simulink model "simulacaoEKF"  (R2016a)
settings: Solver=ode45  StartTime=0.0  StopTime=tf  RelTol=1e-3
undefined symbols (not defined in the file): x0
settings Model: Creator=Davi  LastModifiedBy=davia
settings DataIOCC: LimitDataPoints=on  SaveFormat=Array
settings HardwareCC: ProdBitPerPointer=32  ProdLargestAtomicFloat=None  ProdIntDivRoundTo=Undefined  ProdEndianess=Unspecified  ProdWordSize=32  ProdHWDeviceType=32-bit Generic
settings ModelReferenceCC: PropagateSignalLabelsOutOfModel=off
settings ConfigComp: CovModelRefEnable=Off

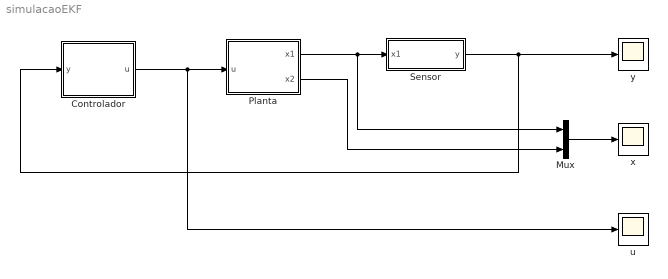
== system simulacaoEKF ==
  Controlador : Subsystem
  Mux : Mux  Inputs=2
  Planta : Subsystem
  "Sensor " : Subsystem
  u : Scope
  x : Scope
  y : Scope
  wires:
  Controlador/1(u) -> u/1, Planta/1(u)
  Planta/1(x1) -> Mux/1, "Sensor "/1(x1)
  "Sensor "/1(y) -> y/1, Controlador/1(y)
  Mux/1 -> x/1
  Planta/2(x2) -> Mux/2

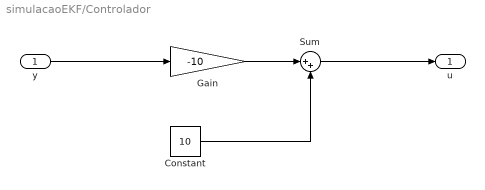
== system simulacaoEKF/Controlador ==
  y : Inport
  Constant : Constant  Value=10
  Gain : Gain  Gain=-10
  Sum : Sum  Inputs=|++
  u : Outport
  wires:
  y/1 -> Gain/1
  Constant/1 -> Sum/2
  Gain/1 -> Sum/1
  Sum/1 -> u/1

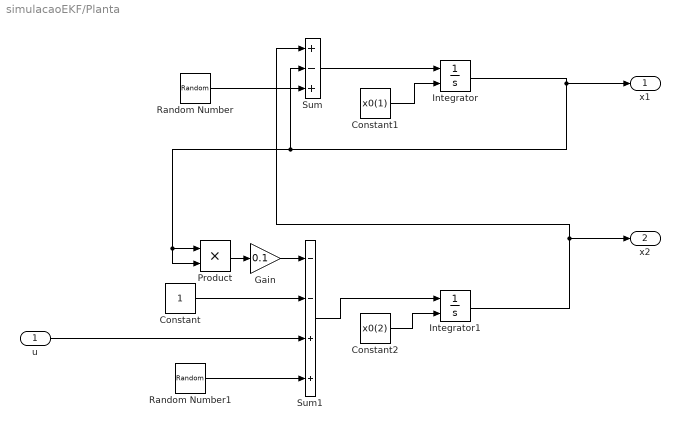
== system simulacaoEKF/Planta ==
  u : Inport
  Constant : Constant
  Constant1 : Constant  Value=x0(1)
  Constant2 : Constant  Value=x0(2)
  Gain : Gain  Gain=0.1
  Integrator : Integrator  InitialConditionSource=external
  Integrator1 : Integrator  InitialConditionSource=external
  Product : Product
  Random Number : RandomNumber  Variance=0.01  Seed=1  SampleTime=0
  Random Number1 : RandomNumber  Variance=0.01  Seed=2  SampleTime=0
  Sum : Sum  Inputs=+-+
  Sum1 : Sum  Inputs=--++
  x1 : Outport
  x2 : Outport  Port=2
  wires:
  Gain/1 -> Sum1/1
  Constant/1 -> Sum1/2
  Sum/1 -> Integrator/1
  Product/1 -> Gain/1
  Integrator1/1 -> x2/1, Sum/1
  Integrator/1 -> x1/1, Sum/2, Product/2, Product/1
  Constant1/1 -> Integrator/2
  Constant2/1 -> Integrator1/2
  Sum1/1 -> Integrator1/1
  u/1 -> Sum1/3
  Random Number/1 -> Sum/3
  Random Number1/1 -> Sum1/4

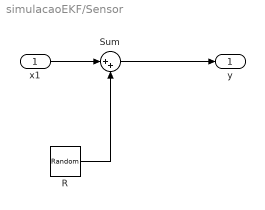
== system simulacaoEKF/Sensor  ==
  x1 : Inport
  R : RandomNumber  Variance=0.01  SampleTime=0
  Sum : Sum  Inputs=|++
  y : Outport
  wires:
  x1/1 -> Sum/1
  R/1 -> Sum/2
  Sum/1 -> y/1
